simulink model "APRV_Bosch"  (R2022b)
settings: Solver=VariableStepAuto  StartTime=0.0  StopTime=100  RelTol=1e-3
undefined symbols (not defined in the file): Charac_Curve, densityHydrogen, hysteresisValve, N2, OperatingTemperature, pinlet, poutlet, responseTimeValve, SpecificGravityHydrogen
libraries: simulink x1
settings Model: Creator=debjani.ghosh  LastModifiedBy=debjani.ghosh
settings DataIOCC: ReturnWorkspaceOutputs=off

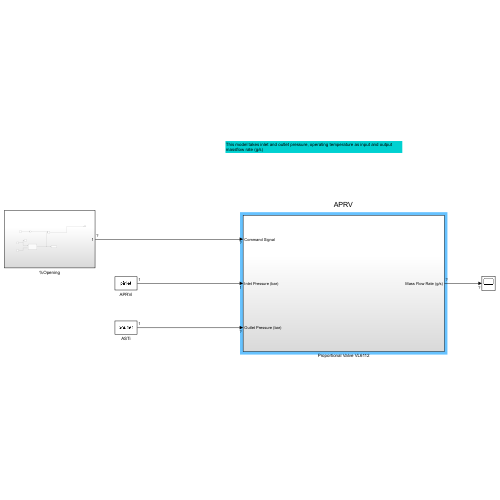
[thumbnail: Simulink's stored preview of the top-level diagram]
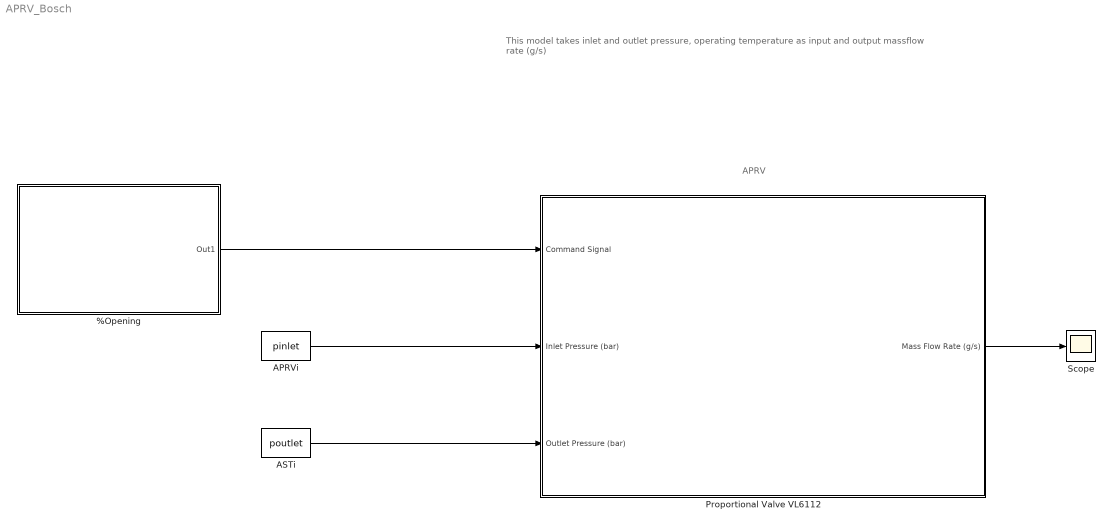
== system APRV_Bosch ==
  note: This model takes inlet and outlet pressure, operating temperature as input and output massflow rate (g/s)
  note: APRV
  %Opening : Subsystem
  APRVi : Constant  Value=pinlet
  ASTi : Constant  Value=poutlet
  Proportional Valve VL6112 : Subsystem
  Scope : Scope
  wires:
  APRVi/1 -> Proportional Valve VL6112/2(Inlet Pressure (bar))
  ASTi/1 -> Proportional Valve VL6112/3(Outlet Pressure (bar))
  Proportional Valve VL6112/1(Mass Flow Rate (g/s)) -> Scope/1
  %Opening/1(Out1) -> Proportional Valve VL6112/1("Command Signal ")

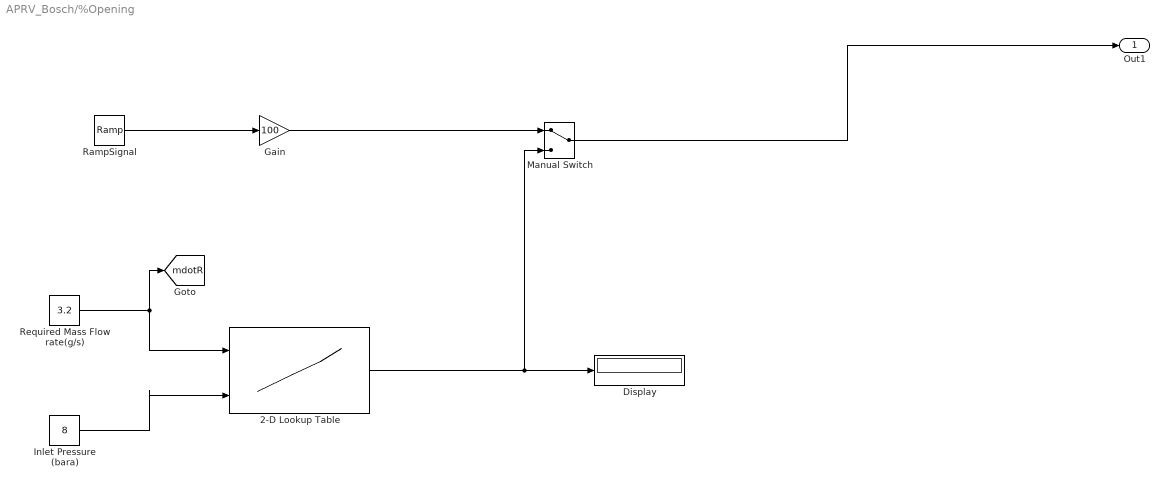
== system APRV_Bosch/%Opening ==
  2-D Lookup Table : Lookup_n-D  BreakpointsForDimension1=[0.1;0.2;0.3;0.4;0.5;0.6;0.7;0.8;0.9;1;1.1;1.2;1.3;1.4;1.5;1.6;1.7;1.8;1.9;2;2.1;2.2;2.3;2.4;2.5;2.6;2.7;2.8;2.9]  BreakpointsForDimension2=[8;10;12;14;16]  Table=Charac_Curve  InternalRulePriority=Speed  RndMeth=Simplest
      settings: InputPortMap=u0,u1
  Display : Display
  Gain : Gain  Gain=100
  Inlet Pressure (bara) : Constant  Value=8
  Manual Switch : ManualSwitch
  RampSignal : simulink/Sources/Ramp  slope=1/100  start=0  InitialOutput=0
  Required Mass Flow rate(g/s) : Constant  Value=3.2
  Out1 : Outport
  tag scope: mdotR=global
  wires:
  Manual Switch/1 -> Out1/1
  2-D Lookup Table/1 -> Manual Switch/2, Display/1
  RampSignal/1 -> Gain/1
  Inlet Pressure (bara)/1 -> 2-D Lookup Table/2
  Required Mass Flow rate(g/s)/1 -> 2-D Lookup Table/1, [mdotR]
  Gain/1 -> Manual Switch/1

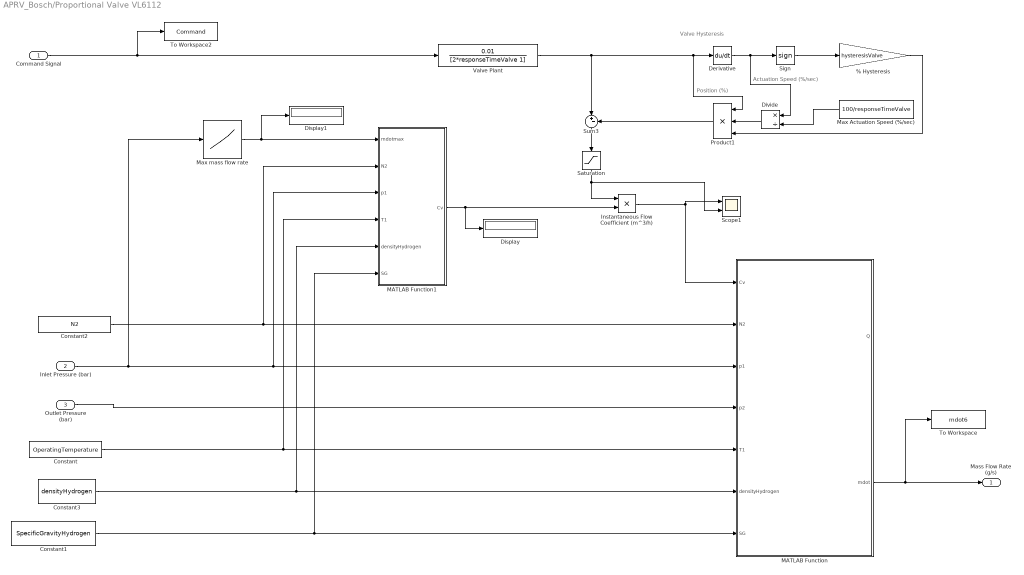
== system APRV_Bosch/Proportional Valve VL6112 ==
  note: Actuation Speed (%/sec)
  note: Position (%)
  note: Valve Hysteresis
  "Command Signal " : Inport
  Inlet Pressure (bar) : Inport  Port=2
  Outlet Pressure (bar) : Inport  Port=3
  % Hysteresis : Gain  Gain=hysteresisValve
  Constant : Constant  Value=OperatingTemperature
  Constant1 : Constant  Value=SpecificGravityHydrogen
  Constant2 : Constant  Value=N2
  Constant3 : Constant  Value=densityHydrogen
  Derivative : Derivative
  Display : Display
  Display1 : Display
  Divide : Product  Inputs=*/
  Instantaneous Flow Coefficient (m^3/h) : Product
  MATLAB Function : MATLAB Function  TreatAsAtomicUnit=on
  MATLAB Function1 : MATLAB Function  TreatAsAtomicUnit=on
  Max Actuation Speed (%/sec) : Constant  Value=100/responseTimeValve
  Max mass flow rate : Lookup_n-D  NumberOfTableDimensions=1  BreakpointsForDimension1=[8,10,12,14,16]  Table=[1.4,1.8,2.2,2.5,2.8]  InternalRulePriority=Speed  RndMeth=Simplest
  Product1 : Product  Inputs=3
  Saturation : Saturate  UpperLimit=1  LowerLimit=0  LinearizeAsGain=off
  Scope1 : Scope  NumInputPorts=2
  Sign : Signum  ZeroCross=off
  Sum3 : Sum  Inputs=|+-
  To Workspace : ToWorkspace  VariableName=mdot6  SaveFormat=Structure With Time  SampleTime=-1
  To Workspace2 : ToWorkspace  VariableName=Command  SaveFormat=Structure With Time  SampleTime=-1
  Valve Plant : TransferFcn  Numerator=0.01  Denominator=[2*responseTimeValve 1]
  Mass Flow Rate (g/s) : Outport
  wires:
  Sign/1 -> % Hysteresis/1
  Derivative/1 -> Divide/1, Sign/1
  % Hysteresis/1 -> Product1/3
  Product1/1 -> Sum3/2
  Sum3/1 -> Saturation/1
  Divide/1 -> Product1/2
  Max Actuation Speed (%/sec)/1 -> Divide/2
  Instantaneous Flow Coefficient (m^3/h)/1 -> MATLAB Function/1(Cv), Scope1/1
  Valve Plant/1 -> Sum3/1, Derivative/1, Product1/1
  "Command Signal "/1 -> To Workspace2/1, Valve Plant/1
  MATLAB Function/2(mdot) -> To Workspace/1, Mass Flow Rate (g/s)/1
  Saturation/1 -> Scope1/2, Instantaneous Flow Coefficient (m^3/h)/1
  Constant1/1 -> MATLAB Function1/6(SG), MATLAB Function/7(SG)
  Constant/1 -> MATLAB Function/5(T1), MATLAB Function1/4(T1)
  Outlet Pressure (bar)/1 -> MATLAB Function/4(p2)
  Constant3/1 -> MATLAB Function1/5(densityHydrogen), MATLAB Function/6(densityHydrogen)
  MATLAB Function1/1(Cv) -> Display/1, Instantaneous Flow Coefficient (m^3/h)/2
  Constant2/1 -> MATLAB Function1/2(N2), MATLAB Function/2(N2)
  Inlet Pressure (bar)/1 -> Max mass flow rate/1, MATLAB Function1/3(p1), MATLAB Function/3(p1)
  Max mass flow rate/1 -> Display1/1, MATLAB Function1/1(mdotmax)

== matlab function APRV_Bosch/Proportional Valve VL6112/MATLAB Function1 ==
  data: mdotmax input; Cv output; N2 input; p1 input; T1 input; densityHydrogen input; SG input
function Cv = fcn(mdotmax,N2, p1,T1,densityHydrogen, SG)

Q = mdotmax /(0.06 * densityHydrogen* 1000/3600);

Cv = Q / (0.471*N2*p1*sqrt(1/(SG*T1)));

== matlab function APRV_Bosch/Proportional Valve VL6112/MATLAB Function ==
  data: Q output; Cv input; N2 input; p1 input; p2 input; T1 input; densityHydrogen input; mdot output; SG input
function [Q,mdot]   = fcn(Cv, N2, p1,p2, T1,densityHydrogen, SG)
%Calculation of mass flow based on Swagelok 
% Valve Sizing Technical Bulletin


%Calculate pressure difference between inlet and outlet

dp = p1-p2;

if p2 > p1/2

     % low pressure drop - subsonic flow

    Q = N2*Cv*p1*(1-(2*dp)/(3*p1))*sqrt(dp/(p1*SG*T1)); % standard volumetric flow rate in lpm 

else
   
    % high pressure drop - sonic flow (independent of downstream pressure)

    Q =  0.471*N2*Cv*p1*sqrt(1/(SG*T1)); % standard volumetric flow rate in lpm  

end

   %Comment: densityHydrogen must be a value dependent on operating T and p

    mdot = 0.06* Q * densityHydrogen* 1000/3600;  %g/s

    %Volumetric flow rate in lpm @ operating T and p
    % T1=T2

   % Vdot = Q * 1.01 * T1 /( p2 * 273);  % lpm
